simulink model "day10p1"  (R2026a)
settings: Solver=FixedStepDiscrete  StopTime=inf
InitFcn:
  | % lmpCntMax = 6;
  | lmpCntMax = 10;
  | % btnCntMax = 10;
  | btnCntMax = 16;
  | % btnStrMax = 39;
  | btnStrMax = 181;
  | lmpStrMax = lmpCntMax + 2;
  | possibilities = dec2bin([0:((2^btnCntMax) - 1)]) - '0';
  | [~, ixs] = sort(sum(possibilities, 2));
  | possibilities = possibilities(ixs, :);
undefined symbols (not defined in the file): DiscIntNeverNeededParam
libraries: simulink x5
(part 1 of 2)
settings Model: PauseTimes=14  Creator=pete  LastModifiedBy=pete

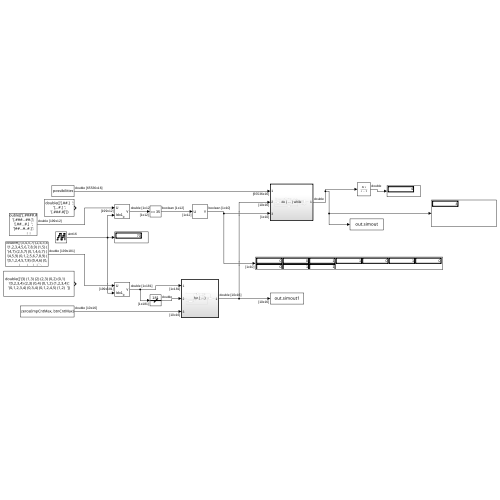
[thumbnail: Simulink's stored preview of the top-level diagram]
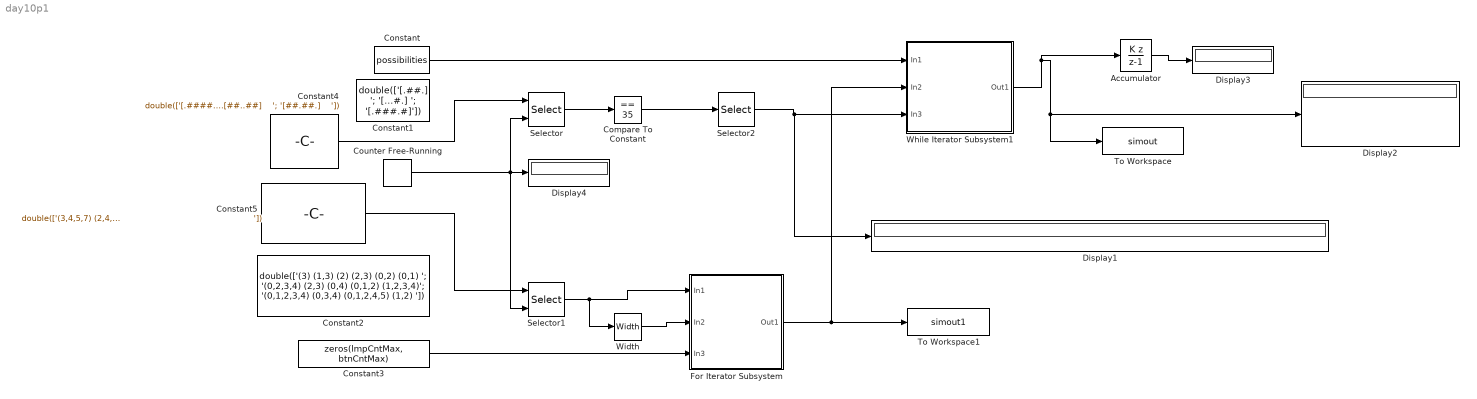
== system day10p1 ==
  Accumulator : DiscreteIntegrator  IntegratorMethod=Accumulation: Backward Euler  SampleTime=-1  ICPrevOutput=DiscIntNeverNeededParam  ICPrevScaledInput=DiscIntNeverNeededParam
  Compare To Constant : simulink/Logic and Bit Operations/Compare To Constant  relop===  const=35  OutDataTypeStr=boolean
  Constant : Constant  Value=possibilities
  Constant1 : Constant  Value=|
      | double(['[.##.]  ';
      | '[...#.] ';
      | '[.###.#]'])
  Constant2 : Constant  Value=|
      | double(['(3) (1,3) (2) (2,3) (0,2) (0,1)        ';
      | '(0,2,3,4) (2,3) (0,4) (0,1,2) (1,2,3,4)';
      | '(0,1,2,3,4) (0,3,4) (0,1,2,4,5) (1,2)  '])
  Constant3 : Constant  Value=zeros(lmpCntMax, btnCntMax)
  Constant4 : Constant  Value=|
      | double(['[.####.#.]  ';
      | '[.###...##.]';
      | '[.##...#.]  ';
      | '[##...#..#.]';
      | '[#...#.#..] ';
      | '[.##...]    ';
      | '[###.....#] ';
      | '[.#.#....]  ';
      | '[###..#..#] ';
      | '[.###]      ';
      | '[...#..#.]  ';
      | '[#.##]      ';
      | '[#####.##.] ';
      | '[.#####]    ';
      | '[.#..###]   ';
      | '[...##.]    ';
      | '[#####.]    ';
      | '[#.##.]     ';
      | '[#....#.##] ';
      | '[.#.#]      ';
      | '[#.#.##.##.]';
      | '[...#]      ';
      | '[..##.#]    ';
      | '[#####.]    ';
      | '[#...#.#]   ';
      | '[##.#..]    ';
      | '[.#..#]     ';
      | '[###.]      ';
      | '[##..#.#..] ';
      | '[###.]      ';
      | '[###.]      ';
      | '[.###]      ';
      | '[##...#.]   ';
      | '[.###.#.]   ';
      | '[#.#...]    ';
      | '[#..##.]    ';
      | '[..##...]   ';
      | '[..#...#]   ';
      | '[.#...##]   ';
      | '[..#..#.#]  ';
      | '[###......] ';
      | '[#.####.]   ';
      | '[..##.##]   ';
      | '[.###]      ';
      | '[.##.#.#..] ';
      | '[#.#.]      ';
      | '[###..#.#]  ';
      | '[#.#..#.]   ';
      | '[#...##]    ';
      | '[...###..]  ';
      | '[####.]     ';
      | '[#...####]  ';
      | '[##.##....#]';
      | '[.#..#]     ';
      | '[#...#....] ';
      | '[.#.....###]';
      | '[..#.#..#]  ';
      | '[#.##..]    ';
      | '[..##...##] ';
      | '[#.#.....#] ';
      | '[.#..##]    ';
      | '[..###]     ';
      | '[.#....#.]  ';
      | '[#.#....###]';
      | '[...#.#.#.] ';
      | '[#..##]     ';
      | '[####]      ';
      | '[..#...##]  ';
      | '[#..#]      ';
      | '[.####.]    ';
      | '[..##.#..##]';
      | '[#.#..##]   ';
      | '[...#..#.]  ';
      | '[#.##...#..]';
      | '[.#..####.#]';
      | '[.#.#]      ';
      | '[##..#.###] ';
      | '[.##.....#.]';
      | '[.....#.#]  ';
      | '[#.#.]      ';
      | '[#.####.###]';
      | '[.##.]      ';
      | '[###..]     ';
      | '[##...#.]   ';
      | '[.#.#.#]    ';
      | '[#...##.]   ';
      | '[###.]      ';
      | '[...#]      ';
      | '[#...#..]   ';
      | '[##..#]     ';
      | '[...#]      ';
      | '[###.]      ';
      | '[#..#####.] ';
      | '[#.#.]      ';
      | '[#...]      ';
      | '[#..##.]    ';
      | '[.#.....]   ';
      | '[###.]      ';
      | '[##...####.]';
      | '[.####.#.#.]';
      | '[.#.##]     ';
      | '[######...] ';
      | '[#..#..#]   ';
      | '[.##...#.]  ';
      | '[...#.#]    ';
      | '[##..#.#.##]';
      | '[....##..]  ';
      | '[####..#.]  ';
      | '[#....#..##]';
      | '[....#]     ';
      | '[.#.#.]     ';
      | '[##...#.#.] ';
      | '[#...#]     ';
      | '[....#]     ';
      | '[###.##..]  ';
      | '[#.#.]      ';
      | '[..#..#]    ';
      | '[#.#.#]     ';
      | '[.#.##]     ';
      | '[.#.#.###..]';
      | '[######..]  ';
      | '[##.##]     ';
      | '[###.##]    ';
      | '[......#..] ';
      | '[##.#.]     ';
      | '[##.#.##..#]';
      | '[.###.]     ';
      | '[..##.###.] ';
      | '[#.#....]   ';
      | '[...#.#..]  ';
      | '[..#.##....]';
      | '[#.##]      ';
      | '[...##]     ';
      | '[#####.#]   ';
      | '[#.##..]    ';
      | '[##..#####] ';
      | '[...##.##.] ';
      | '[.#.#]      ';
      | '[##..]      ';
      | '[.....##..] ';
      | '[###.#..#]  ';
      | '[.##.#.###.]';
      | '[..####]    ';
      | '[#.......##]';
      | '[##.##.]    ';
      | '[###..##]   ';
      | '[####..#.#] ';
      | '[.###..#.#.]';
      | '[.###]      ';
      | '[.....###.#]';
      | '[.###..###.]';
      | '[##.#]      ';
      | '[#.#.]      ';
      | '[.#..#]     ';
      | '[..###]     ';
      | '[.######]   ';
      | '[####...#.] ';
      | '[.#.....#.] ';
      | '[...#.###]  ';
      | '[####]      ';
      | '[#.####..]  ';
      | '[...####]   ';
      | '[#.##.#....]';
      | '[#...###]   ';
      | '[.#.#]      ';
      | '[.##.#.##.] ';
      | '[.##.##.]   ';
      | '[##.#.]     ';
      | '[#.#.]      ';
      | '[#.#.]      ';
      | '[##.###.##.]';
      | '[..##.#.]   ';
      | '[#..##.###.]';
      | '[#......#.] ';
      | '[......#..#]';
      | '[#..#.##]   ';
      | '[...###.]   ';
      | '[..#.#...#.]';
      | '[.#.#.#####]';
      | '[#.#....]   ';
      | '[#.##]      ';
      | '[.#.#.###.#]';
      | '[#.###.]    ';
      | '[#...#.....]';
      | '[.###.##.]  ';
      | '[.....#]    ';
      | '[.####.#..#]';
      | '[.#....]    ';
      | '[.#...]     ';
      | '[#.##.###.#]';
      | '[.###.]     ';
      | '[##.##]     ';
      | '[#.#...##.] ';
      | '[#....##.]  ';
      | '[#.#.###]   ';
      | '[#.##.#..##]';
      | '[##..##.#]  ';
      | '[##..##]    ';
      | '[##.##.]    '])
  Constant5 : Constant  Value=|
      | double(['(3,4,5,7) (2,4,5,6,7) (1,4,7) (1,3,4,7) (1,2,3,4,5,7) (7) (1,2,3,6) (0,1,3,6,7)                                                                                                      ';
      | '(1,2,3,4,5,6,7,8,9) (1,5) (0,1,3,4,5,6,7,8,9) (4,8,9) (0,6,7,9) (1,6,8) (0,1,2,5,6,7,8) (0,1,2,3,5,7,8,9) (1,2,4,5)                                                                  ';
      | '(4,7) (2,5,7) (0,1,4,6,7) (1,4) (0,3,4,5,6,7) (0,1,2,3,4,5,7) (0,1,2,3,4,6) (2,3,5,6,7)                                                                                              ';
      | '(4,5,9) (0,1,2,5,6,7,8,9) (0,1,4,5,6,7,9) (0,1,2,5,6,8) (0,1,2,3,5,7) (1,2,3,4,5,6,8,9) (0,1,3,4,5,6,7,8,9) (3,4,8) (0,4,7,9)                                                        ';
      | '(0,1,2,4,5,7,8) (0,4,6) (0,1,2,7,8) (1,7,8) (1,2,3) (0,5,7,8) (0,1,4,5,6,7) (1,2,5,7,8)                                                                                              ';
      | '(1,3,4) (0,1,3) (3,5) (0) (0,1,2,5) (2,3,4)                                                                                                                                          ';
      | '(0,1,2,3,4,8) (0,3,4,7) (0,1,2,4,5,6,7) (2,3,4) (0,4) (1,2,3,7,8) (0,2,3,6,8) (0,2,4,5,7) (0,1,4,5,6,7,8)                                                                            ';
      | '(1,2,3,4,5,6,7) (1,3) (1,2,3,4,5,7) (1,7) (0,1,2,3,4,6,7) (0,2,4,5,6)                                                                                                                ';
      | '(1,4,5,6) (0,3,7) (1,6,7) (1,2,3,4,8) (0,4,7) (3,4,7) (2,3,5,8)                                                                                                                      ';
      | '(3) (0) (1,3) (1,2) (0,2,3)                                                                                                                                                          ';
      | '(0,2,3,5,6) (1,3,5,6) (5,7) (0,4,7) (1,7) (0,1) (2,4) (0,2,3,4,5,6) (0,3,4,5,6,7) (0)                                                                                                ';
      | '(1,3) (0,3) (0,2,3)                                                                                                                                                                  ';
      | '(1,5,8) (1,2,3,5,6) (2,4,8) (3,4,8) (2,4) (0,1,7,8) (2,3,6) (2,3,7,8) (4,7)                                                                                                          ';
      | '(0,1,3) (0,2) (0,3,4,5) (0,1,4) (0,4)                                                                                                                                                ';
      | '(0,1,4) (1,2) (1,2,3,4,5,6) (0,3,5) (2,3)                                                                                                                                            ';
      | '(2,5) (3) (1,4) (0,1) (0,1,4,5) (4) (2,4,5) (1,2,3,4)                                                                                                                                ';
      | '(0,1,3,4,5) (1,2,3,4) (3) (3,5) (1,5) (0,1,2,4) (2,5) (0,1,2,3)                                                                                                                      ';
      | '(0,1,3,4) (0,1,3) (0,2,3)                                                                                                                                                            ';
      | '(4) (2,3,7) (2,3,4,7,8) (0,1,4,5) (2,3,5,6) (1,2,3,5,6,7,8) (0,3,5,7)                                                                                                                ';
      | '(1,2) (0,2) (0,1,2) (3)                                                                                                                                                              ';
      | '(2,5,6,8) (0,1,2,3,4,5,7,8) (2,7) (0,2,3,6,8) (0,4,6,7,9) (0,1,3,4,5,8,9) (3,4,8) (0,1,5,8)                                                                                          ';
      | '(0,3) (0,2) (1,3) (0,1,3)                                                                                                                                                            ';
      | '(1,3) (0,5) (2,3,4) (0,1,3,4) (1,2,5)                                                                                                                                                ';
      | '(3,4,5) (0,1,2,4,5) (2,3,5) (0,1,5) (1,2,3) (0,2,4,5) (4,5)                                                                                                                          ';
      | '(3,5,6) (0,1,2,5,6) (0,1,2,3,6) (4,6) (2,4,5,6) (0,1,2,3,4) (1,2,3) (0,1,2,4,5) (1,2,3,4,6)                                                                                          ';
      | '(1,2,3,5) (0,3,4,5) (1,2) (0,1,3)                                                                                                                                                    ';
      | '(0,2) (1,4) (0,1,3,4) (0,3,4)                                                                                                                                                        ';
      | '(3) (0) (0,1) (0,1,2) (1,2)                                                                                                                                                          ';
      | '(0,3,4,5,6,7,8) (1,2,4,5,6,7,8) (2,4,7) (0,1,4,6) (1,2,3,4,5,6,7) (1,3,4,5,6) (0,1,3,5,8) (0,1,4,8)                                                                                  ';
      | '(0,1,2) (0,1,3)                                                                                                                                                                      ';
      | '(1,2) (0,2,3) (0,3) (0,1)                                                                                                                                                            ';
      | '(1,2,3) (0,2,3)                                                                                                                                                                      ';
      | '(3,4,6) (1,2,4,5) (0,1,5) (1,6) (0,2,3,5,6)                                                                                                                                          ';
      | '(0,1,2,3,6) (2,3,5,6) (1,2) (3,5) (0,2,4,5,6) (1)                                                                                                                                    ';
      | '(1,4,5) (0,3,4,5) (3,4) (2,5)                                                                                                                                                        ';
      | '(0,1,4,5) (1,2,5) (0,1,2,4) (3,5)                                                                                                                                                    ';
      | '(2,3) (0,1,3,5,6) (2,4) (0,2,3,4,5,6) (0,5)                                                                                                                                          ';
      | '(0,2,6) (1,3) (0,1,2,3,5,6) (1,3,4,5,6) (4,5,6) (1,2,3,4)                                                                                                                            ';
      | '(1,2,4,5) (0,2,3,4,5) (0,2) (0,5) (0,2,4,6) (1,5,6)                                                                                                                                  ';
      | '(1,2,4,7) (1,4,5) (0,1,3,6) (0,1,2,4,6) (2,3,5,7) (0,3,4,5,6,7)                                                                                                                      ';
      | '(0,1,3,4,7) (1,2,3) (1,8) (2,7) (0,1,4,5,7,8) (0,1,3,6,7) (0,1,2,3,4,5,7) (0,1,4,7,8) (0,1,3,4,6,7,8)                                                                                ';
      | '(0,2,3,4,5) (0,1,3,5,6) (0,3,4,5) (0,1,5,6) (2) (1,2,3,4,6) (0,1,3,4,5) (0,1,2,3) (0,6)                                                                                              ';
      | '(2,3) (1,4,5,6) (1,2,3,4,5,6) (0,1,2,5,6) (4,5) (0,1,2,3) (1,4) (0,1,3) (0,5)                                                                                                        ';
      | '(0,1) (2,3) (0,2,3)                                                                                                                                                                  ';
      | '(0,1,4,5,6,7,8) (0,1,3,4,5,6,7) (0,1,2,4,5,7,8) (0,1,2,3,4,6,8) (0,1,3,4,5,7,8) (0,2,3) (5,7)                                                                                        ';
      | '(0,1) (2,3) (1,2) (0,3) (0,2)                                                                                                                                                        ';
      | '(0,1,3,4,6,7) (1,2,3,4,5,7) (0,1,7) (1,4,5,6,7) (0,1,5,7) (5,6,7) (0,4) (1,5) (2,3,4,5) (1,4,7)                                                                                      ';
      | '(1,3,4) (0,1,3) (1,3,4,5,6) (1,2,3,5) (0,2,3,4,5)                                                                                                                                    ';
      | '(0,4,5) (3,4) (0,1,2,3,5) (1,2) (1)                                                                                                                                                  ';
      | '(3,4) (0,2,5,6,7) (0,3,5,6) (0,1,2,3,5,7) (1,2,4,5,7) (0,1,3,4,5) (0,2) (2,6,7) (0,1,4,5,6,7) (2,3,4,5,6,7)                                                                          ';
      | '(4) (0,1,3,4) (2,3,4) (1,2,3) (2) (0,3,4) (2,4)                                                                                                                                      ';
      | '(0,1,3,4) (4,5,6,7) (0,1,2,4,5,6,7) (0) (0,1,2,3,5,7) (0,2,3,7) (1,5) (0,2,3,4,6,7)                                                                                                  ';
      | '(1,5,9) (1,3,5,6,7,8,9) (1,2,4,5,8,9) (1,2,4,5,6,7) (1,3,5,6,7,8) (0,1,2,3,4,5,6,7,9) (0,1,3,4,6,7,8,9) (0,1,5,6,7,9) (2,4,6,7,8)                                                    ';
      | '(0,2,4) (0,2) (0,1,2) (1,4) (2,3,4) (1,2,3,4)                                                                                                                                        ';
      | '(0,1,2,4,8) (0,1,4,5,6,7,8) (3,4,5,6,7,8) (1,3,7,8) (0,2,3,4,8) (2,3) (3,6,7) (0,1,4,5,7) (0,1,5,6) (2,7) (0,6,8)                                                                    ';
      | '(0,1,2,3,5,6,7,8,9) (0,2,3,4,6,7,9) (0,1,2,5,8) (0,1,3,7,8,9) (1,4,5,6,7) (0,1,3,8) (0,1,2,3,5,6,8) (0,1,3,4,5,6,7) (1,2,3,5) (1,3,4,5,6,7,8,9)                                      ';
      | '(0,1,2,3,6) (4,6) (1,2,3,5) (2,3,7) (0,5,6) (0,1,4,6) (0,1,3,5) (1,6,7) (4,7)                                                                                                        ';
      | '(0,1,3,4) (3,4,5) (2,3,4,5) (2,3) (4,5) (1,5)                                                                                                                                        ';
      | '(4,8) (1,4,6,8) (3) (0,1,5) (5,7) (1,2,3,5,7,8) (2,3,4,5) (0) (1,3,4) (0,1,3,4,6,7,8)                                                                                                ';
      | '(6,8) (1,2,3,4,7,8) (1,6,8) (1,2,3,6,7) (1,2,3,5,8) (2,6) (3,4,5,8) (0,2) (1,2,3,4,5,6)                                                                                              ';
      | '(2,4,5) (0,1,3) (4,5) (0,1,5) (0,2,3,4,5)                                                                                                                                            ';
      | '(1,2) (0,1,3) (1,3,4)                                                                                                                                                                ';
      | '(6) (0,4,5) (1,2,4,6) (1,2,3,4,7) (0,1,2,3) (0,1,2,4,5,7) (0,4) (1,7) (0,3,7)                                                                                                        ';
      | '(0,1,2,3,4,5,6,8) (1,3,4,5,7,8,9) (1,2,3,5,6,7,9) (6,8) (6,7) (1,3,5,7,8) (0,1,2,3,6,8,9) (1,2,4,5,6,7,8,9) (0,1,2,3,5,6,8,9) (0,1,4,5,6,7,8,9)                                      ';
      | '(0,1,2,6,7) (0,1,3,4,5,7,8) (1,3,8) (0,1,3,4,6,7,8) (1) (0,2,4,6,7,8) (4) (3,5,7) (0,1,4,8) (1,4,6) (1,2,3,4,7,8)                                                                    ';
      | '(0,1,2,4) (0,3) (0,2,4) (0,2) (1,4)                                                                                                                                                  ';
      | '(0,1,2) (3) (0,3) (0,1,3) (0,1)                                                                                                                                                      ';
      | '(2,3,4,5,6) (0,1,2,3,4,5,7) (0,4,5,6,7) (1,6,7) (0,1,2) (4,5,6,7) (1,3,4,5,6,7)                                                                                                      ';
      | '(0,1) (1,3) (1,2) (3) (0,3) (0,2)                                                                                                                                                    ';
      | '(1,2,4,5) (0,2,3,5) (0,4,5) (0,2)                                                                                                                                                    ';
      | '(2,3,4,5,9) (2,3,4,6,8,9) (0,1,2,3,5,6,7,9) (3,5,6,9) (0,8) (0,3,4,5,6,9) (0,4,8) (1,3,7,8) (1,4,5,7,8) (0,3,4,5) (0,2,3,4,6,7)                                                      ';
      | '(1,2,4,6) (2,5,6) (3,4) (1,3,4,5,6) (0,1,2,4,6) (0,5) (0,1,2,5)                                                                                                                      ';
      | '(1,2,3) (1,4) (0,1,3,4,5,7) (0,7) (1,5) (1,7) (0,2,4,5,6,7) (0,4) (3) (4,5)                                                                                                          ';
      | '(1,2,6,7) (0) (3,4) (0,1,2,5,7,8,9) (7,8) (0,1,2,3,4,6,7,8,9) (6,7,9) (1,2,4,5,7) (0,3,7) (1,3,4,5,6,7,8,9) (1,3,4,6,7,8,9) (0,1,2,4,6)                                              ';
      | '(0,5,7,8) (2,3,4,8,9) (1,2,3,5,8) (0,1,3,4,5,7,8,9) (4,5,6,7,8) (0,2,3,5,8,9) (1,2) (0,1,2,3,6,8) (0,2,4,5,8)                                                                        ';
      | '(1,2) (0,1,3) (2,3)                                                                                                                                                                  ';
      | '(0,2,3,6,7,8) (1,2,5,7) (0,1,2,3,6,7) (2) (0,4,5,8) (1,3,6,7,8) (1,4,5,7,8) (0,2,4,5,6,7) (0,1,2,4,6,7,8) (1,3,5) (1,4,6)                                                            ';
      | '(0,3,7,9) (2,7) (0,2,9) (2,3,8,9) (1,2,3,4,5,7,8,9) (4,7,8) (0,1,3,5,6,7,8) (5,8) (0,2,4,5,6,7,8) (1,7)                                                                              ';
      | '(0,5,7) (0,1,3,4,5,6) (0,1,2,3,6,7) (0,1,2,3) (1,3,4,6,7) (0,4,7) (0) (0,1,3,5,6,7) (1,3,4)                                                                                          ';
      | '(2,3) (0,1,2) (0,2) (0,1) (2)                                                                                                                                                        ';
      | '(0,8,9) (0,2,4,5,6,8,9) (3,4,6,9) (0,1,4,5,6,7,8,9) (1,3,8) (0,2,3,4,5,7,8,9) (0,2,3,6,7) (0,1,2,4,5,6,7,8) (1,6,8)                                                                  ';
      | '(0,3) (2,3) (1,3) (2)                                                                                                                                                                ';
      | '(4) (1) (3,4) (2,3,4) (0,2,3) (0,2)                                                                                                                                                  ';
      | '(0,3) (2,4,5) (0,1,2,4) (0,5,6) (0,2,4,5,6) (1,4,6) (1,2,3)                                                                                                                          ';
      | '(1,4,5) (1,2) (3,4) (0,4,5) (0,2,4) (2,5)                                                                                                                                            ';
      | '(1,2,3,4) (1,2,3,5) (5,6) (4) (0,1,6) (1,3,5,6) (0,2,3,5) (3) (1)                                                                                                                    ';
      | '(0) (0,2,3) (0,1,3) (1,3)                                                                                                                                                            ';
      | '(0,2) (0,1,3) (0,3) (2,3) (1,3) (1,2,3)                                                                                                                                              ';
      | '(4,6) (2,3) (0,2,3,4,5,6) (0,1,2,5) (4,5,6) (1,2,3,5,6) (0,1,3,4,6) (2,3,4,5)                                                                                                        ';
      | '(0,1,2,3) (4) (2,3) (0,3,4) (0,1,4) (0,1) (1,3)                                                                                                                                      ';
      | '(1,2,3) (1) (0,3) (0,2,3) (2)                                                                                                                                                        ';
      | '(0,3) (3) (0,1,2) (0,1) (2,3) (0,2)                                                                                                                                                  ';
      | '(1,2,3,5,6,7,8) (1,3,8) (5,7) (0,1,2,3,4,6,7) (0,1,2,6,7,8) (0,2,3,4,5) (2,3) (1,2,5) (0,7) (0,7,8)                                                                                  ';
      | '(1,2,3) (1,2) (0,1,3)                                                                                                                                                                ';
      | '(2,3) (1,2) (0,1) (1,3) (0,2,3)                                                                                                                                                      ';
      | '(0,1,2,4) (1,3,5) (0,1,4) (1,3)                                                                                                                                                      ';
      | '(1) (0,1,3,4) (1,2,3,4,5,6) (1,5) (1,2,4,5,6) (0,1,2,3,4,6) (0,4,5)                                                                                                                  ';
      | '(1,2) (0,1,2) (1,3) (3) (0) (1)                                                                                                                                                      ';
      | '(1,2,5,6,7,8,9) (2,4,9) (3,4,6,7,8,9) (0,5) (0,1,2,7,9) (0,1,4,5,7,9) (1,3,8) (1,2,3,4,5,6,8,9) (1,2,3,4,6,8,9) (0,1,2,3,4,5,7,8,9) (0,1,3,4,5,6,7) (1,2,4,5,6,7,9) (0,1,2,3,4,5,8,9)';
      | '(0,1,2,4,5,6,7,8) (7,9) (1,2,3,4,5,6,7,8,9) (0,4,5,8) (5) (2,5) (2,3,9) (0,1,3,4,6,7,8) (7,8,9) (3,4) (0,1,3,5,7,8) (1,6,7) (0,1,2,3,4,5,6,8)                                        ';
      | '(0,2) (0,1,2,4) (0,2,3)                                                                                                                                                              ';
      | '(3,4,5) (0,2,4) (0,1,2,3,5,7,8) (2,3) (1,8) (0,1,4,5,6,7,8) (0,4,5,6) (1,2,3,5,6,7,8) (3,4,7) (1,2,4,5,6,7)                                                                          ';
      | '(0,1,2,3,4,5) (0,1,3) (0,6) (0,4) (0,1,2,4,5) (1,2,3,4,5)                                                                                                                            ';
      | '(0,1,3,4,5,6,7) (1,2,5,6) (0,3,6) (0,6,7) (1,2,4,5,7) (2,3,5,6) (1,2,4,7)                                                                                                            ';
      | '(1,5) (1,3,4,5) (2,3,4,5) (0,1,2,3) (4) (2,3)                                                                                                                                        ';
      | '(1,3,4,5,6,7,9) (0,7) (0,1,2,3,6,8,9) (0,1,4,5,7,8,9) (4,5) (3,4,8) (0,1,3,6,8) (0,2,3,4,5,6,7) (1,3,8) (0,1,2,4,5,7,8,9)                                                            ';
      | '(2,3,4,5) (4,5) (1,2,3,4,5,7) (1,2,7) (0,1,2,3) (0,1,3,4,6)                                                                                                                          ';
      | '(0,1,3,6) (0,1,2,5,6) (1,5) (0,3,5,6,7) (0,3,4,6,7) (1,2,3,4,6,7) (0,1,2,3,6,7)                                                                                                      ';
      | '(0,1,3,5,7,8) (1,2,3,6,9) (2,4,5,7,8) (0,1,2,6,7,8,9) (0,5,7) (1,2,6,7) (1,4) (5,8) (3) (4,5,7,8,9) (3,6)                                                                            ';
      | '(0,1,3) (2,3) (0,1,3,4)                                                                                                                                                              ';
      | '(0,4) (1,4) (0,2,4) (3,4)                                                                                                                                                            ';
      | '(0,1,4,5,6,8) (0,1,2,3,6,8) (0,4,5,6,7) (0,2,3,4,7) (0,2,3,6,8) (0,1,2,5,6,7,8) (1,3,7) (1,2,6)                                                                                      ';
      | '(0,1,3) (2,3) (1,3,4)                                                                                                                                                                ';
      | '(2,3,4) (0,1,3) (0,2) (2) (1,2,3) (3,4) (0,1,2)                                                                                                                                      ';
      | '(0,1,2,4,7) (2,3) (1,3,5,7) (0,1,2,3,7) (0,3,4,6) (0,1,7) (0,1,2,5,6,7) (0,1,2,7) (5,7) (2,6,7)                                                                                      ';
      | '(1,2,3) (0,2)                                                                                                                                                                        ';
      | '(2,3,5) (0,1,3,4) (2,5) (1,3,5) (1,5) (0,2) (0,2,3,5)                                                                                                                                ';
      | '(1,2) (3) (1) (4) (1,3,4) (0,2) (0,2,4)                                                                                                                                              ';
      | '(2,3) (0,2) (0,3,4) (0,1,2,3) (0,1,2)                                                                                                                                                ';
      | '(0,3,4,5,6,7,9) (1,2,4,5,6,7,8) (4,5) (0,1,2,4,5,6,7,8) (0,1,4,5,6,8) (0,3,4,5,7,8,9) (1,6) (5,6,8) (1,4,6,8,9) (0,1,6) (0,1,2,4,5,7,8,9)                                            ';
      | '(1,2,3,5,6,7) (0,1,3,6) (5,6) (0,2,3,7) (0,1,3,4,5) (0,1,2,3,4,5) (2,3,4,5,6) (0,1,2,4,5)                                                                                            ';
      | '(0,1,2,3) (2,4) (0,1,2) (0,2,4) (1,3)                                                                                                                                                ';
      | '(0,2,3,4,5) (1,5) (0,1) (0,2,4) (2,3,4,5) (0,3,5) (0,3)                                                                                                                              ';
      | '(0,2,3,4,6,7,8) (0,1,2,3,4,6,7) (1) (0,3,4,5,6,7) (0,1,2,3,4,5,6,8) (3,4,7) (0,1,2,3,5,7,8) (4,6,7) (5,6,7) (4,5,6,8) (1,4,6,7)                                                      ';
      | '(0,1,4) (1,3,4) (0,1,2) (0,3) (0,2)                                                                                                                                                  ';
      | '(0,1,4,5,6,7,8,9) (0,2,4,5,6,7,8,9) (1,3,5,8) (0,2,5,9) (2,4,6,7,8) (1,5,9) (2,4,5,6,9) (0,2,4,8) (0,2,3,4,5,7,8,9) (0,1,2,3,4,5,6,7) (1,2,4,5,7,8,9) (2,4,7,8,9)                    ';
      | '(1,3,4) (1,2,3,4) (0,1) (2,3,4) (1,2) (0,1,2,4)                                                                                                                                      ';
      | '(0,1,2,3,4,6,7,8) (1,4,8) (0,1,3,5,7,8) (0,2,3,4,6,8) (0,1,2,6,7,8) (2,3,4,5,6) (1,2,3,5,6,7,8)                                                                                      ';
      | '(1,2,5) (0,1,2,5) (0,2,4,5) (1,2,4) (0,3,4) (0,2) (0,3,4,6)                                                                                                                          ';
      | '(1,4,5,6,7) (3,4) (0,1,2,3,6,7) (1,2,3,4,7) (0,2) (3,5) (3,4,6) (0,1,2,4,5,7)                                                                                                        ';
      | '(0,3,6,9) (4,8) (0,1,3,4,5,6,7,8) (2,8,9) (1,2,3,4,5,6,9) (2,3,4,6,7,8) (3,5,6,7) (0,2,3,5,7,9) (0,1,5) (0,1,5,6,8,9) (2,4,5,8,9) (1,2,3,5,6,7) (0,2,3,5,6,7,8,9)                    ';
      | '(0,2,3) (0,1,3)                                                                                                                                                                      ';
      | '(2,4) (0,1,4) (0,1,3)                                                                                                                                                                ';
      | '(3,4) (1,3,5,6) (1,2) (0,3,4) (5,6) (2,3,4,5,6) (0,1,6) (0,1,2,6)                                                                                                                    ';
      | '(0,2) (1,2,3,4) (1,3) (2,3,5) (0,1,3,4) (0,1,4) (0,2,3,5) (1,3,4,5)                                                                                                                  ';
      | '(0,1,2,4,5,7,8) (0,6,8) (1,2,5,6,8) (0,1,2,3,5) (0,1,4,6,7,8) (4,5,6) (1,3,4,5,7) (1,3,6,7) (2,4,6,7) (1,2,5,6,7,8)                                                                  ';
      | '(1,2,5,6,8) (0,5,8) (3,5,7,8) (3,7) (0,1,2,3,4,5,6,8) (0,4,7) (4,5,6,8) (0,1,2,4,5,7,8)                                                                                              ';
      | '(1,3) (0,2)                                                                                                                                                                          ';
      | '(0,1,3) (2,3) (0,3) (0,2,3) (1)                                                                                                                                                      ';
      | '(0,4,8) (0,1,2,3,5,7) (0,3,4,7) (4,5,6,7,8) (3,5,6) (0,3,6) (0,1,3,4,5,6,7,8) (0,1,5,6) (0,7) (0,3,4,6,7) (0,1,2,4,5,6,8)                                                            ';
      | '(1,2,3) (1,3,5,6,7) (2,4,5) (0,1,4,5,7) (0,2,3,4,5,7) (0,1,2,4,5,6) (0,2,3,5,7)                                                                                                      ';
      | '(0,2,3,7,8,9) (2,3,6,9) (0,1,3,5,7,9) (1,2,3,5,6,7,9) (0,4,5,6,7,8) (2,3,5,6,7) (0,2,3,5,7,9) (1,9) (0,1,2,3,4,6,7,9) (4,8) (0,1,3,4,5,6,8,9)                                        ';
      | '(1,3) (0,2,3,5) (0,1,2,4) (0,2,4,5) (0,1,2,3) (4,5) (2,4) (2,3,4)                                                                                                                    ';
      | '(0,3,5,8) (3,5,6,7,9) (0,2,3,4,5,7,8,9) (5,6,7,9) (1,2,3,4,6,7,8,9) (1,3,4,5,7) (2,4,6,7,8,9) (4,6,8,9) (2,5,6) (2,4,5,6,7,9) (1,2,5,8,9)                                            ';
      | '(0,1,2,4,5) (3,5) (0,1,2,5) (1,2,4,5) (0,1,3,4) (0,3,5) (1,4,5)                                                                                                                      ';
      | '(5) (1,2,4,5) (1,2,4,6) (0,2,4) (0,1,2,3,4,6) (0,1,3,5,6) (0,3,4)                                                                                                                    ';
      | '(0,3,4,6,7) (0,2,4,6) (0,1,2,3,6,8) (1,3,4,5,6,7,8) (1,2,8) (2,3) (5,6,8)                                                                                                            ';
      | '(4,5) (5,7) (0,5,6,8,9) (0,1,5,6,9) (0,1,2,4,5,6,7,8) (3,4) (0,1,3,4,6,7,8,9) (1,4,5,6,7,8,9)                                                                                        ';
      | '(0,2) (1,2,3)                                                                                                                                                                        ';
      | '(8) (1,3,4,6,7,9) (0) (1,2,4,5,6,7,8) (0,1,2,3,6,7) (2,4) (1,5) (1,2,6,8,9) (5,7) (0,2,4,5,8) (0,1,2,3,4,6,7,9) (1,2,3,5,7,8,9)                                                      ';
      | '(9) (0,1,2,6,8) (2,3,6,7,8) (0,5) (0,1,3,5,6,7,8,9) (2,3,4) (1,2,4,5,6,8,9) (2,4,5,7,8) (1,3,5,6,7,8,9) (4,6,9) (0,7) (1,9) (1,2,3,6,8)                                              ';
      | '(1,3) (0,1,3) (1,2)                                                                                                                                                                  ';
      | '(0,2) (1,3) (1) (0,2,3)                                                                                                                                                              ';
      | '(2) (0,1,2,3) (1,4) (0,2,3,4)                                                                                                                                                        ';
      | '(1,2,4) (0,2,4) (1,4) (1,2,3,4) (2,3,4) (0,2,3,4)                                                                                                                                    ';
      | '(1,2,3,4,5) (0,1,3,4,6) (1,2,4,5,6) (0,1,5,6) (0,3) (1,5,6) (0,2) (0,1,2,5,6)                                                                                                        ';
      | '(0,1,2,4,5) (1,2,3,8) (0,2,3,7,8) (0,1,2,3,4,7) (0,1,3,4,6,7,8) (0,2,4,7,8) (0,1,2,3,8) (1,3,5,6,8) (1,2,3,4,5) (0,4,5,7) (2,8)                                                      ';
      | '(0,1,4) (0,1,2,3,4,6,7,8) (3,4,5,6,7) (0,2) (0,2,3,8) (2,3,5,7) (0,1,4,5,7) (0,2,3,4,5,6,7,8)                                                                                        ';
      | '(0,1,2,3,6,7) (3,6,7) (0,3,7) (3,4) (2,3,4,6,7) (0,1,5,6) (1,2,3,4,6) (1,4,5) (0,2,5,6)                                                                                              ';
      | '(0,2) (0,3) (1,3)                                                                                                                                                                    ';
      | '(0,1,3,4,5,6) (1,2,3,5) (0,1,3,5,7) (0,1,2,4,5,6) (1,2,6,7) (1,2,3,4,5,6)                                                                                                            ';
      | '(1,2,3,5,6) (0,3) (4,5) (0,3,6) (0,1,2) (0,3,5) (1,2,4,6) (3,4,6)                                                                                                                    ';
      | '(0,1,2,3,5,6,7,9) (0,4,5,6,8,9) (4,5,6,7) (0,2,3,4,5,6,8) (2,3,4,5,6,9) (0,1,2,4,5,7,8,9) (0,3,4,5,6,8,9) (1,3,6,7,8) (4,6,8) (5,7) (5) (7,8,9)                                      ';
      | '(0,1,3,4,6) (0,2,3,5,6) (2,3,4,6) (1,6) (1,2,3,5,6) (0,6) (2,6)                                                                                                                      ';
      | '(1,3) (0,2,3)                                                                                                                                                                        ';
      | '(2,8) (0,3,4,5,6,7) (1,5,7) (1,2,3,4,6,7,8) (0,1,5,6,7,8) (7) (1,2,3,5,7,8) (2,3,4,6,8) (0,1,2,3,4,7,8) (1,3,4,6,7)                                                                  ';
      | '(0,2,4,5) (1,3,4) (0,1,3,6) (1,2,3,5,6) (1,2,5)                                                                                                                                      ';
      | '(0,3,4) (1,2,4) (0,1,3,4) (2)                                                                                                                                                        ';
      | '(0,2) (0,1,3) (0,2,3) (1,3) (0,3)                                                                                                                                                    ';
      | '(1,3) (0,2)                                                                                                                                                                          ';
      | '(0,1,2,3,4,5,6,9) (0,1,2,4,5,7,8,9) (0,1,7,8) (1,2,3,4,6,7,8,9) (2,3,4,9) (0,1,2,4,6,7,8) (0,1,2,6,9) (3,4,6,7,9)                                                                    ';
      | '(0,4,6) (1,3,6) (1,2,3,5,6) (2,4,5,6) (0,1) (0,2,3,5) (2,3,5)                                                                                                                        ';
      | '(0,1,2,3,4,5,7,8) (4,6) (1,4,5,8) (0,2,3,5,6,7,8,9) (0,3,4,5,7,9) (0,2,5,6) (2,4) (1,9) (0,1,2,3,4,5,7,8,9) (0,1,3,4,6,7,8,9)                                                        ';
      | '(0,3) (0,2,5,6,7) (0,1,3,4,5) (1,2,8) (0,2,3,5,6,7,8) (2,3,6,7) (0,1,2,4,5,6,7,8) (0,2,3,4,5,7,8)                                                                                    ';
      | '(6,9) (1,2,4,5) (0,1,2,3,4,5,6,7,9) (1,2,4,5,7,8,9) (1,3,4,5,7,8) (0,5,6) (1,2,4,5,6,7,8) (0,1,3,4,6,7,8,9) (0,2,3,7,8,9) (3,4,5,6) (1,2,3)                                          ';
      | '(2) (2,4) (0,1,2,3,6) (4,5) (3,6) (3) (0,5) (0,1,3,4,6) (0,2,3,6)                                                                                                                    ';
      | '(1,6) (0,6) (1,2,3,5) (3,4,5) (0,1,2,5,6) (0,2,3,4,5)                                                                                                                                ';
      | '(0,1,2,3,4,5,6,8,9) (1,2,3,4,5,6,7) (1,6,7,8) (4,6) (3,7,9) (0,1,2,3,5,6,9) (2,3,4,7,8) (0,2,4,6,7,8,9)                                                                              ';
      | '(1,2,3,8) (0,3,4,5,6,7,8,9) (2,3,6,7,9) (1,3,4,6,7) (1,5,6) (4,5,8,9) (9) (1,3,4,6,8,9) (1,2,3,6,7,8) (4,5,6,7) (1,2,4,6,8,9) (0,1,7,9)                                              ';
      | '(3) (0,2,3,4,5) (0,2,5) (0,1,2,3,4) (0,1,2,4,5) (0,1,2,3,4,5) (0,1,2,5) (0,2,3,5,6) (3,5)                                                                                            ';
      | '(2) (3) (0) (1) (0,3) (2,3)                                                                                                                                                          ';
      | '(0,1,2,3,4,7,8,9) (0,1,3,4,5,6,8,9) (0,1,3,4,5,6,7,8) (0,1,2,3,4,5,6,8) (0,1,6,7,8,9) (2,7,9) (0,1,3,5,9) (2,5,7,8,9) (1,3,5,6,7,9) (8,9) (3,7) (7)                                  ';
      | '(1,2,3,5) (2) (0,2,3,4) (1,2,3,4) (2,5) (1,2,4,5) (1,3,4) (1,4)                                                                                                                      ';
      | '(0,1,2,3,6,8,9) (1,2,3,6) (1,2,3,4,5,8) (1,2,3,5,6,9) (1,3,4,5,6,7) (2,3,4,5,7,8,9) (0,2,3,5,7,8,9) (0,1,2,4,5,7,8,9) (0,1,3,4,5,6,7,9) (6,7,8) (0,3,4,5,6,7,8,9) (0,2,5,8,9) (3,6)  ';
      | '(0,1,2,3,5,6) (0,1,2,3,4,6) (0,4,6) (0,7) (2,3,4,6,7) (0,5) (0,2,3,4,5,6) (1,3,4,7) (0,2,5) (0,1,2,3,6,7)                                                                            ';
      | '(2,4,5) (2,4) (0,2,3) (1,3) (1,3,4,5) (0,1) (0,2,3,5)                                                                                                                                ';
      | '(3,4,5,7) (0,1,2,5,6,8) (0,2,4,5) (0,2,4,7) (0,1,4,6,7,8,9) (0,1,2,3,4,6,8) (0,1,2,3,5,6,8) (0,2,3,5) (0,1,2,4,5,6,7) (0,3,4,9)                                                      ';
      | '(4,5) (0,2,3) (0,2,4,5) (1,3) (1,2,3,4)                                                                                                                                              ';
      | '(0,2) (3) (1) (1,3) (0,3) (1,4)                                                                                                                                                      ';
      | '(0,2,3,5,6,7,9) (0,4,5,6,7,8,9) (4,7,9) (4,5,6) (2,5) (0,2,6,9) (0,1,2,3,4,5,6,7) (0,1,6,8,9) (1,3,5,6,7,8,9)                                                                        ';
      | '(1,2) (0,3,4) (1,2,3) (0,4)                                                                                                                                                          ';
      | '(2,3) (2) (0,3,4) (1,2)                                                                                                                                                              ';
      | '(0,1,4,5,7,8) (0,1,3,4,5,7) (1,2,3,6,7,8) (2,4,7) (1,2,4,5,6,7,8) (0,1,2,5,6,8) (1,2,4,5,6,8) (0,1,3,5,6,7,8) (0,3,5)                                                                ';
      | '(0,2,3,4,5,6) (5) (2,3) (1,2,3,4,5) (0,1,2) (0,3,6,7) (1,5) (2,3,5,7) (4,6)                                                                                                          ';
      | '(0,3) (0,1,2,5) (1,2,3) (2,3,6) (1,4,5) (0,2,4,5,6) (1,3,4,5,6)                                                                                                                      ';
      | '(1,4,6,8) (0,1,3,4,8,9) (0,2,3,5,8,9) (1,2,3,4,6,7,8,9) (0,1,2,3,4,5,7,8,9) (2,6,7,8,9) (0,1,2,6,7,8) (1,4,5,9) (1,3,4,5,6,8)                                                        ';
      | '(0,2,5) (1,5) (1,3,4,5,6,7) (2,6) (0,2,3,4,5,6,7) (0,2,7) (3,7) (4,6) (0,2,5,6,7)                                                                                                    ';
      | '(0,3,4) (2) (0,1,2,4) (0,1,2,5) (0,2,3)                                                                                                                                              ';
      | '(3,4,5) (2,4,5) (0,2,4) (1,2) (1,2,3,5) (2,3) (2,3,4,5)                                                                                                                              '])
  Counter Free-Running : simulink/Sources/Counter Free-Running  NumBits=16  tsamp=-1
  Display{1..4} (4 alike) : Display
  For Iterator Subsystem : Subsystem  TreatAsAtomicUnit=on
  Selector : Selector  NumberOfDimensions=2  IndexMode=Zero-based  InputPortWidth=3  IndexOptions=Index vector (port),Select all  Indices=[1 3],1  OutputSizes=1,1  RuntimeRangeChecks=on
  Selector1 : Selector  NumberOfDimensions=2  IndexMode=Zero-based  InputPortWidth=3  IndexOptions=Index vector (port),Select all  Indices=[1 3],1  OutputSizes=1,1  RuntimeRangeChecks=on
  Selector2 : Selector  IndexMode=Zero-based  InputPortWidth=lmpStrMax  IndexOptions=Index vector (dialog)  Indices=[1:lmpCntMax]  OutputSizes=1  RuntimeRangeChecks=on
  To Workspace : ToWorkspace  VariableName=simout  SaveFormat=Timeseries  SampleTime=-1
  To Workspace1 : ToWorkspace  VariableName=simout1  SaveFormat=Timeseries  SampleTime=-1
  While Iterator Subsystem1 : Subsystem  TreatAsAtomicUnit=on
  Width : Width
  wires:
  Constant4/1 -> Selector/1
  Constant5/1 -> Selector1/1
  Selector/1 -> Compare To Constant/1
  Compare To Constant/1 -> Selector2/1
  Selector1/1 -> Width/1, For Iterator Subsystem/1(In1)
  Width/1 -> For Iterator Subsystem/2(In2)
  For Iterator Subsystem/1(Out1) -> To Workspace1/1, While Iterator Subsystem1/2(In2)
  Selector2/1 -> Display1/1, While Iterator Subsystem1/3(In3)
  While Iterator Subsystem1/1(Out1) -> Accumulator/1, To Workspace/1, Display2/1
  Constant/1 -> While Iterator Subsystem1/1(In1)
  Accumulator/1 -> Display3/1
  Constant3/1 -> For Iterator Subsystem/3(In3)
  Counter Free-Running/1 -> Selector1/2, Selector/2, Display4/1

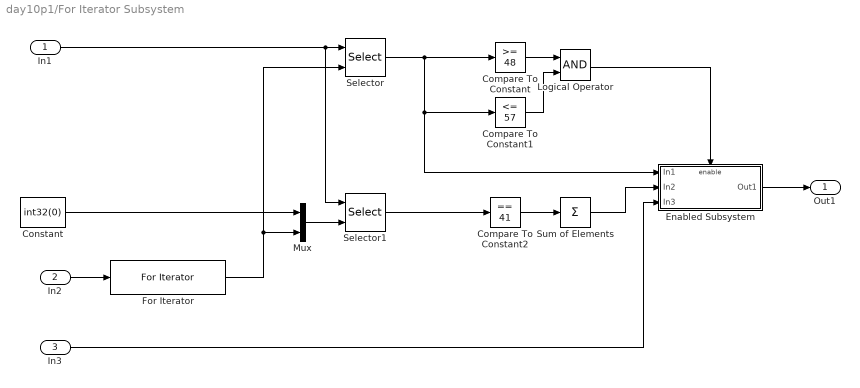
== system day10p1/For Iterator Subsystem ==
  In1 : Inport
  In2 : Inport  Port=2
  In3 : Inport  Port=3
  Compare To Constant : simulink/Logic and Bit Operations/Compare To Constant  relop=>=  const=48  OutDataTypeStr=boolean
  Compare To Constant1 : simulink/Logic and Bit Operations/Compare To Constant  relop=<=  const=57  OutDataTypeStr=boolean
  Compare To Constant2 : simulink/Logic and Bit Operations/Compare To Constant  relop===  const=41  OutDataTypeStr=boolean
  Constant : Constant  Value=int32(0)
  Enabled Subsystem : Subsystem  TreatAsAtomicUnit=on
  For Iterator : ForIterator  ResetStates=reset  IterationSource=external  IndexMode=Zero-based
  Logical Operator : Logic  AllPortsSameDT=off  OutDataTypeStr=boolean
  Mux : Mux  Inputs=2
  Selector : Selector  IndexMode=Zero-based  InputPortWidth=btnStrMax  IndexOptions=Index vector (port)  Indices=[1 3]  OutputSizes=1  RuntimeRangeChecks=on
  Selector1 : Selector  IndexMode=Zero-based  InputPortWidth=btnStrMax  IndexOptions=Starting and ending indices (port)  Indices=[1 3]  OutputSizes=1  RuntimeRangeChecks=on
  Sum of Elements : Sum  Inputs=+
  Out1 : Outport
  wires:
  In2/1 -> For Iterator/1
  Constant/1 -> Mux/1
  For Iterator/1 -> Selector/2, Mux/2
  In1/1 -> Selector1/1, Selector/1
  Mux/1 -> Selector1/2
  Selector/1 -> Enabled Subsystem/1(In1), Compare To Constant1/1, Compare To Constant/1
  Compare To Constant/1 -> Logical Operator/1
  Compare To Constant1/1 -> Logical Operator/2
  Selector1/1 -> Compare To Constant2/1
  Compare To Constant2/1 -> Sum of Elements/1
  Logical Operator/1 -> Enabled Subsystem/Enable
  Enabled Subsystem/1(Out1) -> Out1/1
  Sum of Elements/1 -> Enabled Subsystem/2(In2)
  In3/1 -> Enabled Subsystem/3(In3)

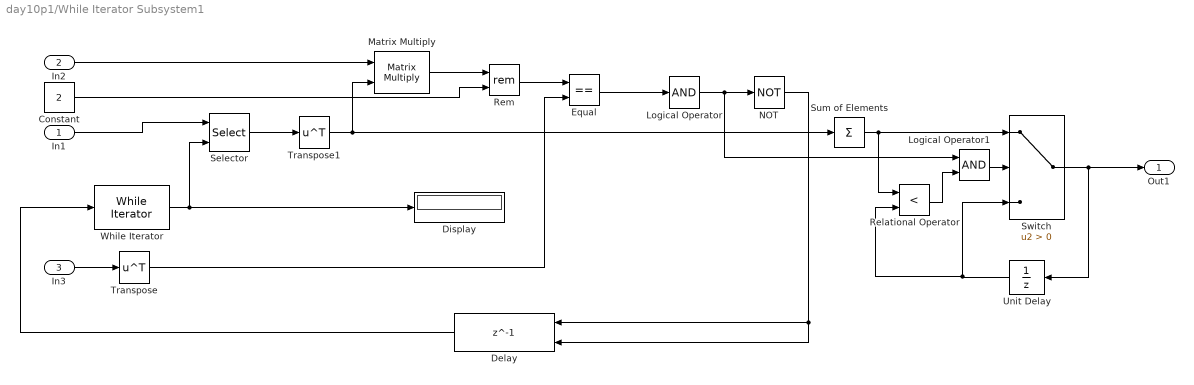
== system day10p1/While Iterator Subsystem1 ==
  In1 : Inport
  In2 : Inport  Port=2
  In3 : Inport  Port=3
  Constant : Constant  Value=2
  Delay : Delay  DelayLength=1  InitialConditionSource=Input port
      settings: InputPortMap=u0,p4
  Display : Display
  Equal : RelationalOperator  Operator===  OutDataTypeStr=boolean  RndMeth=Simplest  InputSameDT=off
  Logical Operator : Logic  Inputs=1  AllPortsSameDT=off  OutDataTypeStr=boolean
  Logical Operator1 : Logic  AllPortsSameDT=off  OutDataTypeStr=boolean
  Matrix Multiply : Product  Multiplication=Matrix(*)
  NOT : Logic  Operator=NOT  IconShape=distinctive  AllPortsSameDT=off  OutDataTypeStr=boolean
  Relational Operator : RelationalOperator  Operator=<  OutDataTypeStr=boolean  RndMeth=Simplest  InputSameDT=off
  Rem : Math  Operator=rem
  Selector : Selector  NumberOfDimensions=2  InputPortWidth=3  IndexOptions=Index vector (port),Select all  Indices=[1 3],1  OutputSizes=1,1  RuntimeRangeChecks=on
  Sum of Elements : Sum  Inputs=+
  Switch : Switch  Criteria=u2 > Threshold  SaturateOnIntegerOverflow=off  InputSameDT=off
  Transpose : Math  Operator=transpose
  Transpose1 : Math  Operator=transpose
  Unit Delay : UnitDelay  InitialCondition=Inf  SampleTime=-1
  While Iterator : WhileIterator  MaxIters=-1  WhileBlockType=do-while  ResetStates=reset  ShowIterationPort=on
  Out1 : Outport
  wires:
  In3/1 -> Transpose/1
  In1/1 -> Selector/1
  While Iterator/1 -> Display/1, Selector/2
  Selector/1 -> Transpose1/1
  In2/1 -> Matrix Multiply/1
  Transpose1/1 -> Sum of Elements/1, Matrix Multiply/2
  Matrix Multiply/1 -> Rem/1
  Constant/1 -> Rem/2
  Rem/1 -> Equal/1
  Transpose/1 -> Equal/2
  Equal/1 -> Logical Operator/1
  Logical Operator/1 -> Logical Operator1/1, NOT/1
  NOT/1 -> Delay/2, Delay/1
  Delay/1 -> While Iterator/1
  Switch/1 -> Out1/1, Unit Delay/1
  Sum of Elements/1 -> Relational Operator/1, Switch/1
  Logical Operator1/1 -> Switch/2
  Relational Operator/1 -> Logical Operator1/2
  Unit Delay/1 -> Switch/3, Relational Operator/2
